simulink model "spectrum_analyser"  (R2020a)
settings: Solver=VariableStepAuto  StartTime=0.0  StopTime=100000/256e6  RelTol=1e-3
InitFcn:
  | fs = 256e6;
undefined symbols (not defined in the file): designMultirateFIR
libraries: hdlsllib x14, dspmlti4 x6, dspswit3 x4, simulink x3, dspsigops x2, dspsigattribs x2, slib_spectrum_analyser x1
(part 1 of 2)
settings Model: Creator=david  LastModifiedBy=kevin
settings OptimizationCC: BlockReduction=off  ConditionallyExecuteInputs=off  DefaultParameterBehavior=Inlined
settings DebuggingCC: AlgebraicLoopMsg=error
settings HardwareCC: ProdBitPerPointer=32  ProdBitPerSizeT=32  ProdBitPerPtrDiffT=32  ProdLargestAtomicFloat=None  ProdIntDivRoundTo=Undefined  ProdEndianess=Unspecified  ProdWordSize=32  ProdHWDeviceType=ASIC/FPGA->ASIC/FPGA  TargetBitPerPointer=64  TargetBitPerSizeT=64  TargetBitPerPtrDiffT=64  TargetLongLongMode=on  TargetIntDivRoundTo=Zero  TargetEndianess=LittleEndian  TargetWordSize=64  TargetHWDeviceType=Custom Processor->MATLAB Host Computer  ProdEqTarget=off

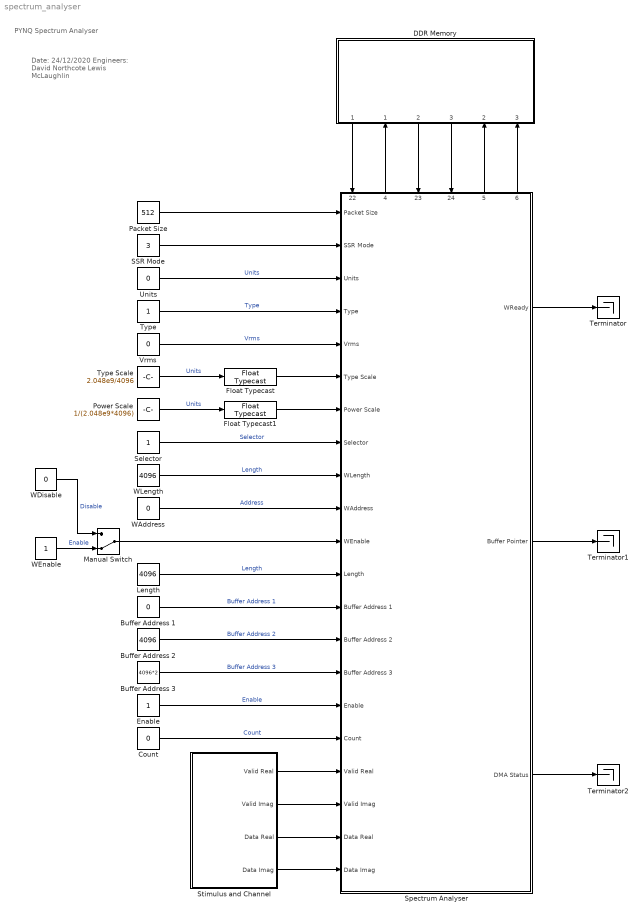
== system spectrum_analyser ==
  note: Date:		24/12/2020
      | Engineers:	David Northcote
      | 			Lewis McLaughlin
  note: PYNQ Spectrum Analyser
  Buffer Address 1 : Constant  Value=0  OutDataTypeStr=uint32  SampleTime=1/fs
  Buffer Address 2 : Constant  Value=4096  OutDataTypeStr=uint32  SampleTime=1/fs
  Buffer Address 3 : Constant  Value=4096*2  OutDataTypeStr=uint32  SampleTime=1/fs
  Count : Constant  Value=0  OutDataTypeStr=uint32  SampleTime=1/fs
  DDR Memory : Subsystem
      settings: PortSchema="{\"entries\":[{\"content\":{\"sides\":[{\"content\":{\"connectorIds\":[]},\"type\":\"ConnectorPlacement.EquallySpacedRectSide\",\"uuid\":\"d9e4a1d3-1a90-455f-8481-c9ba23695512\"},{\"content\":{\"connectorIds\":[],\"side\":\"RIGHT\"},\"type\":\"ConnectorPlacement.EquallySpacedRectSide\",\"uuid\":\"d5cbf6c4-ca28-4b6e-a385-26c8d45a1027\"},{\"content\":{\"connectorIds\":[],\"side\":\"TOP\"},\"type\":\"ConnectorPlacement.EquallySpacedRectSide\",\"uuid\":\"1f61d25a-c781-4c7b-9600-adf853a1e7e2\"},{\"content\":{\"connectorIds\":[\"Out1\",\"In1\",\"Out2\",\"Out3\",\"In2\",\"In3\"],\"side\":\"BOTTOM\"},\"type\":\"ConnectorPlacement.EquallySpacedRectSide\",\"uuid\":\"b1131089-25c6-4639-a5ae-8f8dd9cc5fb0\"}]},\"type\":\"ConnectorPlacement.EquallySpacedConnector\",\"uuid\":\"baa6cdf8-4ad4-4b76-ad8b-23012dfe0a1e\"}],\"packageUris\":[\"http://schema.mathworks.com/mf0/Connector/19700101\"],\"version\":\"1.0\"}"
  Enable : Constant  OutDataTypeStr=uint32  SampleTime=1/fs
  Float Typecast : FloatTypecast
  Float Typecast1 : FloatTypecast
  Length : Constant  Value=4096  OutDataTypeStr=uint32  SampleTime=1/fs
  Manual Switch : ManualSwitch  CurrentSetting=0
  Packet Size : Constant  Value=512  OutDataTypeStr=uint32  SampleTime=-1
  Power Scale : Constant  Value=1/(2.048e9*4096)  OutDataTypeStr=single  SampleTime=-1
  SSR Mode : Constant  Value=3  OutDataTypeStr=uint32  SampleTime=-1
  Selector : Constant  OutDataTypeStr=uint32  SampleTime=-1
  Spectrum Analyser : Subsystem  TreatAsAtomicUnit=on
      settings: PortSchema="{\"entries\":[{\"content\":{\"sides\":[{\"content\":{\"connectorIds\":[\"In1\",\"In2\",\"In3\",\"In4\",\"In5\",\"In6\",\"In7\",\"In8\",\"In9\",\"In10\",\"In11\",\"In12\",\"In13\",\"In14\",\"In15\",\"In16\",\"In17\",\"In18\",\"In19\",\"In20\",\"In21\"]},\"type\":\"ConnectorPlacement.EquallySpacedRectSide\",\"uuid\":\"cc2cc642-11de-4ac0-af05-03fa45094956\"},{\"content\":{\"connectorIds\":[\"Out1\",\"Out2\",\"Out3\"],\"side\":\"RIGHT\"},\"type\":\"ConnectorPlacement.EquallySpacedRectSide\",\"uuid\":\"6db9fe89-3396-451d-908f-f3a7c837a938\"},{\"content\":{\"connectorIds\":[\"In22\",\"Out4\",\"In23\",\"In24\",\"Out5\",\"Out6\"],\"side\":\"TOP\"},\"type\":\"ConnectorPlacement.EquallySpacedRectSide\",\"uuid\":\"bd53c193-ffde-49a5-ab31-00011bb85ae9\"}]},\"type\":\"ConnectorPlacement.EquallySpacedConnector\",\"uuid\":\"7a597bb5-a924-4306-9058-810ed9aba18e\"}],\"packageUris\":[\"http://schema.mathworks.com/mf0/Connector/19700101\"],\"version\":\"1.0\"}"
  Stimulus and Channel : Subsystem
  Terminator : Terminator
  Terminator1 : Terminator
  Terminator2 : Terminator
  Type : Constant  OutDataTypeStr=uint32  SampleTime=-1
  Type Scale : Constant  Value=2.048e9/4096  OutDataTypeStr=single  SampleTime=-1
  Units : Constant  Value=0  OutDataTypeStr=uint32  SampleTime=-1
  Vrms : Constant  Value=0  OutDataTypeStr=uint32  SampleTime=-1
  WAddress : Constant  Value=0  OutDataTypeStr=uint32  SampleTime=1/fs
  WDisable : Constant  Value=0  OutDataTypeStr=uint32  SampleTime=1/fs
  WEnable : Constant  OutDataTypeStr=uint32  SampleTime=1/fs
  WLength : Constant  Value=4096  OutDataTypeStr=uint32  SampleTime=1/fs
  wires:
  Stimulus and Channel/1(Valid Real) -> Spectrum Analyser/18(Valid Real)
  Stimulus and Channel/2(Valid Imag) -> Spectrum Analyser/19(Valid Imag)
  Stimulus and Channel/3(Data Real) -> Spectrum Analyser/20(Data Real)
  Stimulus and Channel/4(Data Imag) -> Spectrum Analyser/21(Data Imag)
  Vrms/1 -> Spectrum Analyser/5(Vrms)  "Vrms"
  Type/1 -> Spectrum Analyser/4(Type)  "Type"
  Units/1 -> Spectrum Analyser/3(Units)  "Units"
  Type Scale/1 -> Float Typecast/1  "Units"
  Float Typecast/1 -> Spectrum Analyser/6(Type Scale)
  Float Typecast1/1 -> Spectrum Analyser/7(Power Scale)
  Power Scale/1 -> Float Typecast1/1  "Units"
  Selector/1 -> Spectrum Analyser/8(Selector)  "Selector"
  SSR Mode/1 -> Spectrum Analyser/2(SSR Mode)
  Packet Size/1 -> Spectrum Analyser/1(Packet Size)
  WEnable/1 -> Manual Switch/2  "Enable"
  WDisable/1 -> Manual Switch/1  "Disable"
  Manual Switch/1 -> Spectrum Analyser/11(WEnable)
  WAddress/1 -> Spectrum Analyser/10(WAddress)  "Address"
  WLength/1 -> Spectrum Analyser/9(WLength)  "Length"
  Spectrum Analyser/4(axim_rd_m2s) -> DDR Memory/1(axim_rd_m2s)
  Spectrum Analyser/5(axim_wr_m2s) -> DDR Memory/2(axim_wr_m2s)
  Spectrum Analyser/6(axim_wr_data) -> DDR Memory/3(axim_wr_data)
  DDR Memory/1(axim_rd_s2m) -> Spectrum Analyser/22(axim_rd_s2m)
  DDR Memory/2(axim_rd_data) -> Spectrum Analyser/23(axim_rd_data)
  DDR Memory/3(axim_wr_s2m) -> Spectrum Analyser/24(axim_wr_s2m)
  Length/1 -> Spectrum Analyser/12(Length)  "Length"
  Buffer Address 1/1 -> Spectrum Analyser/13(Buffer Address 1)  "Buffer Address 1"
  Buffer Address 3/1 -> Spectrum Analyser/15(Buffer Address 3)  "Buffer Address 3"
  Buffer Address 2/1 -> Spectrum Analyser/14(Buffer Address 2)  "Buffer Address 2"
  Enable/1 -> Spectrum Analyser/16(Enable)  "Enable"
  Count/1 -> Spectrum Analyser/17(Count)  "Count"
  Spectrum Analyser/1(WReady) -> Terminator/1
  Spectrum Analyser/2(Buffer Pointer) -> Terminator1/1
  Spectrum Analyser/3(DMA Status) -> Terminator2/1

== system spectrum_analyser/DDR Memory ==
  axim_rd_m2s : Inport
  axim_wr_m2s : Inport  Port=2
  axim_wr_data : Inport  Port=3
  AXI Read Interface Response Model : Subsystem
      settings: PortSchema="{\"entries\":[{\"content\":{\"sides\":[{\"content\":{\"connectorIds\":[]},\"type\":\"ConnectorPlacement.EquallySpacedRectSide\",\"uuid\":\"2b557e1e-8026-43d3-80e6-d6d80e534d60\"},{\"content\":{\"connectorIds\":[\"Out1\",\"In1\",\"Out2\"],\"side\":\"RIGHT\"},\"type\":\"ConnectorPlacement.EquallySpacedRectSide\",\"uuid\":\"d37ff7b5-bcab-46eb-bf2f-7b890d421095\"},{\"content\":{\"connectorIds\":[],\"side\":\"TOP\"},\"type\":\"ConnectorPlacement.EquallySpacedRectSide\",\"uuid\":\"b7392330-958c-44c2-9b9d-e2e6efc00005\"}]},\"type\":\"ConnectorPlacement.EquallySpacedConnector\",\"uuid\":\"d6fedbd7-9a1a-42de-85f8-78943e8230da\"}],\"packageUris\":[\"http://schema.mathworks.com/mf0/Connector/19700101\"],\"version\":\"1.0\"}"
  AXI Write Interface Response Model : Subsystem
      settings: PortSchema="{\"entries\":[{\"content\":{\"sides\":[{\"content\":{\"connectorIds\":[]},\"type\":\"ConnectorPlacement.EquallySpacedRectSide\",\"uuid\":\"6953abbe-a6d5-4686-b276-b89fe5e6bb23\"},{\"content\":{\"connectorIds\":[],\"side\":\"RIGHT\"},\"type\":\"ConnectorPlacement.EquallySpacedRectSide\",\"uuid\":\"539ff6ac-c243-4534-87d0-888ff9534a8b\"},{\"content\":{\"connectorIds\":[],\"side\":\"TOP\"},\"type\":\"ConnectorPlacement.EquallySpacedRectSide\",\"uuid\":\"8a126ba7-8eec-4733-ae4d-1ac2504ae558\"},{\"content\":{\"connectorIds\":[\"Out1\",\"In1\",\"In2\"],\"side\":\"BOTTOM\"},\"type\":\"ConnectorPlacement.EquallySpacedRectSide\",\"uuid\":\"05254abb-7168-4864-8cc1-53a55061df5a\"}]},\"type\":\"ConnectorPlacement.EquallySpacedConnector\",\"uuid\":\"821e8dd7-bdc5-437f-b697-1dcc78127ace\"}],\"packageUris\":[\"http://schema.mathworks.com/mf0/Connector/19700101\"],\"version\":\"1.0\"}"
  axim_rd_s2m : Outport
  axim_rd_data : Outport  Port=2
  axim_wr_s2m : Outport  Port=3
  wires:
  axim_wr_m2s/1 -> AXI Write Interface Response Model/1(axim_wr_m2s)
  AXI Read Interface Response Model/1(axim_rd_data) -> axim_rd_data/1  "axim_rd_data"
  AXI Write Interface Response Model/1(axim_wr_s2m) -> axim_wr_s2m/1
  axim_rd_m2s/1 -> AXI Read Interface Response Model/1(axim_rd_m2s)
  AXI Read Interface Response Model/2(axim_rd_s2m) -> axim_rd_s2m/1  "axim_rd_s2m"
  axim_wr_data/1 -> AXI Write Interface Response Model/2(axim_wr_data)

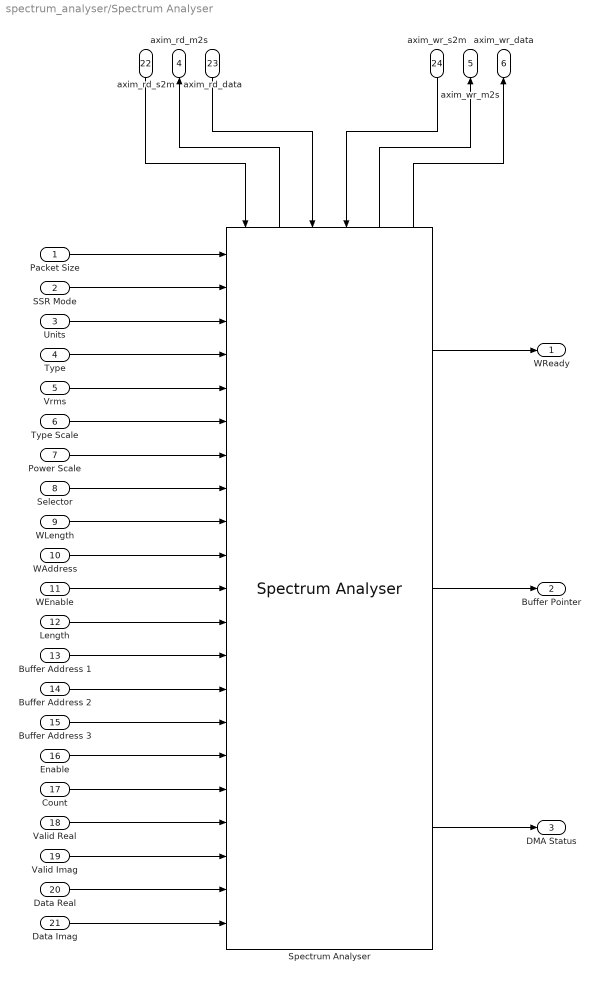
== system spectrum_analyser/Spectrum Analyser ==
  Packet Size : Inport
  SSR Mode : Inport  Port=2
  Units : Inport  Port=3
  Type : Inport  Port=4
  Vrms : Inport  Port=5
  Type Scale : Inport  Port=6
  Power Scale : Inport  Port=7
  Selector : Inport  Port=8
  WLength : Inport  Port=9
  WAddress : Inport  Port=10
  WEnable : Inport  Port=11
  Length : Inport  Port=12
  Buffer Address 1 : Inport  Port=13
  Buffer Address 2 : Inport  Port=14
  Buffer Address 3 : Inport  Port=15
  Enable : Inport  Port=16
  Count : Inport  Port=17
  Valid Real : Inport  Port=18
  Valid Imag : Inport  Port=19
  Data Real : Inport  Port=20
  Data Imag : Inport  Port=21
  axim_rd_s2m : Inport  Port=22
  axim_rd_data : Inport  Port=23
  axim_wr_s2m : Inport  Port=24
  Spectrum Analyser : slib_spectrum_analyser/Spectrum Analyser  SystemSampleTime=-1  Latency=0  AutoFrameSizeCalculation=off
      settings: PortSchema="{\"entries\":[{\"content\":{\"sides\":[{\"content\":{\"connectorIds\":[\"In1\",\"In2\",\"In3\",\"In4\",\"In5\",\"In6\",\"In7\",\"In8\",\"In9\",\"In10\",\"In11\",\"In12\",\"In13\",\"In14\",\"In15\",\"In16\",\"In17\",\"In18\",\"In19\",\"In20\",\"In21\"]},\"type\":\"ConnectorPlacement.EquallySpacedRectSide\",\"uuid\":\"d853649d-72ce-4bc9-937e-6765c6958e4b\"},{\"content\":{\"connectorIds\":[\"Out1\",\"Out2\",\"Out3\"],\"side\":\"RIGHT\"},\"type\":\"ConnectorPlacement.EquallySpacedRectSide\",\"uuid\":\"8ee09e61-17e3-46fa-8063-dedf2b48f93c\"},{\"content\":{\"connectorIds\":[\"In22\",\"Out4\",\"In23\",\"In24\",\"Out5\",\"Out6\"],\"side\":\"TOP\"},\"type\":\"ConnectorPlacement.EquallySpacedRectSide\",\"uuid\":\"c9845971-679e-4c10-9868-9337bdd39c3c\"}]},\"type\":\"ConnectorPlacement.EquallySpacedConnector\",\"uuid\":\"5955e85d-b605-4825-a1fe-b5d4f394d259\"}],\"packageUris\":[\"http://schema.mathworks.com/mf0/Connector/19700101\"],\"version\":\"1.0\"}"
  WReady : Outport
  Buffer Pointer : Outport  Port=2
  DMA Status : Outport  Port=3
  axim_rd_m2s : Outport  Port=4
  axim_wr_m2s : Outport  Port=5
  axim_wr_data : Outport  Port=6
  wires:
  Packet Size/1 -> Spectrum Analyser/1
  SSR Mode/1 -> Spectrum Analyser/2
  Units/1 -> Spectrum Analyser/3
  Type/1 -> Spectrum Analyser/4
  Vrms/1 -> Spectrum Analyser/5
  Type Scale/1 -> Spectrum Analyser/6
  Power Scale/1 -> Spectrum Analyser/7
  Selector/1 -> Spectrum Analyser/8
  WLength/1 -> Spectrum Analyser/9
  WAddress/1 -> Spectrum Analyser/10
  WEnable/1 -> Spectrum Analyser/11
  Length/1 -> Spectrum Analyser/12
  Buffer Address 1/1 -> Spectrum Analyser/13
  Buffer Address 2/1 -> Spectrum Analyser/14
  Buffer Address 3/1 -> Spectrum Analyser/15
  Enable/1 -> Spectrum Analyser/16
  Count/1 -> Spectrum Analyser/17
  Valid Real/1 -> Spectrum Analyser/18
  Valid Imag/1 -> Spectrum Analyser/19
  Data Real/1 -> Spectrum Analyser/20
  Data Imag/1 -> Spectrum Analyser/21
  axim_rd_s2m/1 -> Spectrum Analyser/22
  axim_rd_data/1 -> Spectrum Analyser/23
  axim_wr_s2m/1 -> Spectrum Analyser/24
  Spectrum Analyser/1 -> WReady/1
  Spectrum Analyser/2 -> Buffer Pointer/1
  Spectrum Analyser/3 -> DMA Status/1
  Spectrum Analyser/4 -> axim_rd_m2s/1
  Spectrum Analyser/5 -> axim_wr_m2s/1
  Spectrum Analyser/6 -> axim_wr_data/1

== system spectrum_analyser/Stimulus and Channel ==
  Channel : Subsystem
  Enable : Constant  OutDataTypeStr=boolean  SampleTime=-1
  Transmitter : Subsystem  TreatAsAtomicUnit=on
  Value : Constant  Value=hex2dec('7FFF7FFF')  OutDataTypeStr=uint32  SampleTime=-1
  Valid Real : Outport
  Valid Imag : Outport  Port=2
  Data Real : Outport  Port=3
  Data Imag : Outport  Port=4
  wires:
  Enable/1 -> Transmitter/1(Enable)  "Enable"
  Transmitter/1(Valid) -> Channel/1(Valid)
  Transmitter/2(Data) -> Channel/2(Data)
  Value/1 -> Transmitter/2(Value)  "Value"
  Channel/3(Valid Imag) -> Valid Imag/1
  Channel/4(Data Imag) -> Data Imag/1
  Channel/1(Valid Real) -> Valid Real/1
  Channel/2(Data Real) -> Data Real/1

== system spectrum_analyser/DDR Memory/AXI Read Interface Response Model ==
  axim_rd_m2s : Inport
  Bus Creator : BusCreator  Inputs=2
  Bus Selector : BusSelector  OutputSignals=rd_addr,rd_len,rd_avalid
  Constant3 : Constant  OutDataTypeStr=boolean  SampleTime=-1
  DDR : Subsystem  mask{DDR_DATA=uint16(ones(1,4096)*2^15)}
      mask init:
      | %load('ram_data');
  axim_rd_data : Outport  VectorParamsAs1DForOutWhenUnconnected=off
  axim_rd_s2m : Outport  Port=2  VectorParamsAs1DForOutWhenUnconnected=off
  wires:
  Bus Selector/2 -> DDR/2(rd_len)  "<rd_len>"
  DDR/2(rd_aready) -> Bus Creator/1  "rd_aready"
  Bus Selector/3 -> DDR/3(rd_avalid)  "<rd_avalid>"
  axim_rd_m2s/1 -> Bus Selector/1
  Bus Selector/1 -> DDR/1(rd_addr)  "<rd_addr>"
  Constant3/1 -> DDR/4(rd_ready)
  DDR/3(rd_dvalid) -> Bus Creator/2  "rd_dvalid"
  DDR/1(rd_data) -> axim_rd_data/1  "rd_data"
  Bus Creator/1 -> axim_rd_s2m/1

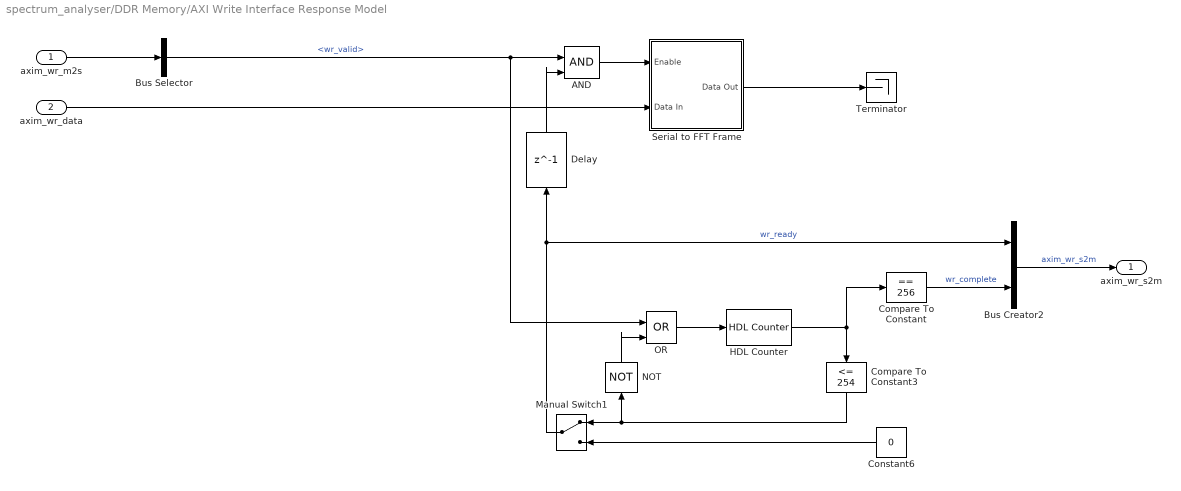
== system spectrum_analyser/DDR Memory/AXI Write Interface Response Model ==
  axim_wr_m2s : Inport
  axim_wr_data : Inport  Port=2
  AND : Logic  IconShape=distinctive  AllPortsSameDT=off  OutDataTypeStr=boolean
  Bus Creator2 : BusCreator  Inputs=2
  Bus Selector : BusSelector  OutputSignals=wr_valid
  Compare To Constant : simulink/Logic and Bit Operations/Compare To Constant  relop===  const=256  OutDataTypeStr=boolean
  Compare To Constant3 : simulink/Logic and Bit Operations/Compare To Constant  relop=<=  const=254  OutDataTypeStr=boolean
  Constant6 : Constant  Value=0  OutDataTypeStr=boolean  SampleTime=-1
  Delay : Delay  DelayLength=1  InitialCondition=0  UseCircularBuffer=on
  HDL Counter : hdlsllib/Sources/HDL Counter  CountType=Count limited  CountInit=0  CountStep=1  CountMax=256  CountFromType=Initial value  CountFrom=0  CountResetPort=off  CountLoadPort=off  CountEnbPort=on  CountDirPort=off  CountDataType=Unsigned  CountWordLen=10  CountFracLen=0  CountSampTime=1
  Manual Switch1 : ManualSwitch
  NOT : Logic  Operator=NOT  IconShape=distinctive  AllPortsSameDT=off  OutDataTypeStr=boolean
  OR : Logic  Operator=OR  IconShape=distinctive  AllPortsSameDT=off  OutDataTypeStr=boolean
  Serial to FFT Frame : Subsystem  mask{N=4096}
      mask prompts: N "FFT Size:"
      mask DialogControl DescGroupVar Prompt: Serial to FFT Frame
      mask DialogControl DescTextVar Prompt: This block converts serial FFT data to a frame of FFT data. An FFT shift is applied to correct for out of order FFT data.
      mask DialogControl ParameterGroupVar Prompt: Main
  Terminator : Terminator
  axim_wr_s2m : Outport
  wires:
  Delay/1 -> AND/2
  Compare To Constant/1 -> Bus Creator2/2  "wr_complete"
  Bus Selector/1 -> AND/1, OR/1  "<wr_valid>"
  AND/1 -> Serial to FFT Frame/1(Enable)
  Constant6/1 -> Manual Switch1/2
  HDL Counter/1 -> Compare To Constant3/1, Compare To Constant/1
  Compare To Constant3/1 -> NOT/1, Manual Switch1/1
  OR/1 -> HDL Counter/1
  NOT/1 -> OR/2
  Bus Creator2/1 -> axim_wr_s2m/1  "axim_wr_s2m"
  Manual Switch1/1 -> Bus Creator2/1, Delay/1  "wr_ready"
  axim_wr_m2s/1 -> Bus Selector/1
  Serial to FFT Frame/1(Data Out) -> Terminator/1
  axim_wr_data/1 -> Serial to FFT Frame/2(Data In)

== system spectrum_analyser/Stimulus and Channel/Channel ==
  Valid : Inport
  Data : Inport  Port=2
  RF-ADC : Subsystem  mask{fs_ghz=4.096, decim=2x, ssr=8, mode=Fine, fc=0.256, fph=0, fcoarse=fs/4}
      mask prompts: fs_ghz "Sample Rate (GHz):"; decim "Interpolation Mode:"; ssr "Samples per AXI4-Stream Cycle:"; mode "Mixer Type:"; fc "NCO Frequency (GHz):"; fph "NCO Phase (Rads):"; fcoarse "Frequency:"
      mask init:
      | % Obtain the sample rate in Hz
      | fs = str2double(get_param(gcb, 'fs_ghz'))*1e9;
      | 
      | % Set the mode of the RF-DAC interpolation filter
      | switch get_param(gcb, 'decim')
      |     case '1x'
      |         D = 1;
      |     case '2x'
      |         D = 2;
      |     case '4x'
      |         D = 4;
      |     case '8x'
      |         D = 8;
      |     otherwise
      |         D = 1;
      | end
      | 
      | % Get the AXI-Stream clock for display to user
      | axi_clk = (fs/(str2double(get_param(gcb, 'ssr'))*D))*1e-6;
      | 
      | % Get the block mask object to manipulate settings
      | mo = get_param(gcb, 'MaskObject');
      | 
      | % Update text to display the required AXI-Stream clock
      | tc = mo.getDialogControl('axi_text');
      | tc.Prompt = ['      Required AXI-Stream Clock: ', num2str(axi_clk), ' MHz'];
      | 
      | % Set the RF-DAC Mixer mode
      | switch get_param(gcb, 'mode')
      |     case 'Bypass'
      |         m = 0;
      |     case 'Coarse'
      |         m = 1;
      |     case 'Fine'
      |         m = 2;
      |     otherwise
      |         m = 0;
      | end
      | 
      | % Set the RF-DAC Coarse Mixer mode
      | switch get_param(gcb, 'fcoarse')
      |     case 'fs/2'
      |         mc = 0;
      |     case 'fs/4'
      |         mc = 1;
      |     case '-fs/4'
      |         mc = 2;
      |     otherwise
      |         mc = 0;
      | end
      | 
      | % Set other blocks
      | set_param([gcb, '/Decimation Filter'], 'decim', get_param(gcb, 'decim'));
      mask Callback fs_ghz:
      | % Obtain the sample rate in Hz
      | fs = str2double(get_param(gcb, 'fs_ghz'))*1e9;
      | 
      | % Set the mode of the RF-DAC interpolation filter
      | switch get_param(gcb, 'decim')
      |     case '1x'
      |         D = 1;
      |     case '2x'
      |         D = 2;
      |     case '4x'
      |         D = 4;
      |     case '8x'
      |         D = 8;
      |     otherwise
      |         D = 1;
      | end
      | 
      | % Get the AXI-Stream clock for display to user
      | axi_clk = (fs/(str2double(get_param(gcb, 'ssr'))*D))*1e-6;
      | 
      | % Get the block mask object to manipulate settings
      | mo = get_param(gcb, 'MaskObject');
      | 
      | % Update text to display the required AXI-Stream clock
      | tc = mo.getDialogControl('axi_text');
      | tc.Prompt = ['      Required AXI-Stream Clock: ', num2str(axi_clk), ' MHz'];
      mask TypeOptions decim: 1x | 2x | 4x | 8x
      mask Callback decim:
      | % Obtain the sample rate in Hz
      | fs = str2double(get_param(gcb, 'fs_ghz'))*1e9;
      | 
      | % Set the mode of the RF-DAC interpolation filter
      | switch get_param(gcb, 'decim')
      |     case '1x'
      |         D = 1;
      |     case '2x'
      |         D = 2;
      |     case '4x'
      |         D = 4;
      |     case '8x'
      |         D = 8;
      |     otherwise
      |         D = 1;
      | end
      | 
      | % Get the AXI-Stream clock for display to user
      | axi_clk = (fs/(str2double(get_param(gcb, 'ssr'))*D))*1e-6;
      | 
      | % Get the block mask object to manipulate settings
      | mo = get_param(gcb, 'MaskObject');
      | 
      | % Update text to display the required AXI-Stream clock
      | tc = mo.getDialogControl('axi_text');
      | tc.Prompt = ['      Required AXI-Stream Clock: ', num2str(axi_clk), ' MHz'];
      mask TypeOptions ssr: 1 | 2 | 3 | 4 | 5 | 6 | 7 | 8 | 9 | 10 | 11 | 12 | 13 | 14 | 15 | 16
      mask Callback ssr:
      | % Obtain the sample rate in Hz
      | fs = str2double(get_param(gcb, 'fs_ghz'))*1e9;
      | 
      | % Set the mode of the RF-DAC interpolation filter
      | switch get_param(gcb, 'decim')
      |     case '1x'
      |         D = 1;
      |     case '2x'
      |         D = 2;
      |     case '4x'
      |         D = 4;
      |     case '8x'
      |         D = 8;
      |     otherwise
      |         D = 1;
      | end
      | 
      | % Get the AXI-Stream clock for display to user
      | axi_clk = (fs/(str2double(get_param(gcb, 'ssr'))*D))*1e-6;
      | 
      | % Get the block mask object to manipulate settings
      | mo = get_param(gcb, 'MaskObject');
      | 
      | % Update text to display the required AXI-Stream clock
      | tc = mo.getDialogControl('axi_text');
      | tc.Prompt = ['      Required AXI-Stream Clock: ', num2str(axi_clk), ' MHz'];
      mask TypeOptions mode: Coarse | Fine
      mask Callback mode:
      | % Get the block mask object to manipulate settings
      | mo = get_param(gcb, 'MaskObject');
      | 
      | % Hide group depending on Mixer mode choice
      | switch get_param(gcb, 'mode')
      |     case 'Bypass'
      |         mo.getDialogControl('coarse_group').Visible='off';
      |         mo.getDialogControl('mixer_group').Visible='off';
      |     case 'Coarse'
      |         mo.getDialogControl('coarse_group').Visible='on';
      |         mo.getDialogControl('mixer_group').Visible='off';
      |     case 'Fine'
      |         mo.getDialogControl('coarse_group').Visible='off';
      |         mo.getDialogControl('mixer_group').Visible='on';
      |     otherwise
      |         mo.getDialogControl('coarse_group').Visible='off';
      |         mo.getDialogControl('mixer_group').Visible='off';
      | end
      mask TypeOptions fcoarse: fs/2 | fs/4 | -fs/4
      mask DialogControl DescGroupVar Prompt: RF-DAC
      mask DialogControl DescTextVar Prompt: This block simulates one RF-ADC channel.
      mask DialogControl main_group Prompt: Data Settings
      mask DialogControl axi_text Prompt: Required AXI-Stream Clock: 256 MHz
      mask DialogControl Container5 Prompt: Mixer Settings
  RF-DAC : Subsystem  mask{fs_ghz=4.096, interp=4x, ssr=4, mode=Fine, fc=0.512, fph=0, fcoarse=fs/4}
      mask prompts: fs_ghz "Sample Rate (GHz):"; interp "Interpolation Mode:"; ssr "Samples per AXI4-Stream Cycle:"; mode "Mixer Type:"; fc "NCO Frequency (GHz):"; fph "NCO Phase (Rads):"; fcoarse "Frequency:"
      mask init:
      | % Obtain the sample rate in Hz
      | fs = str2double(get_param(gcb, 'fs_ghz'))*1e9;
      | 
      | % Set the mode of the RF-DAC interpolation filter
      | switch get_param(gcb, 'interp')
      |     case '1x'
      |         L = 1;
      |     case '2x'
      |         L = 2;
      |     case '4x'
      |         L = 4;
      |     case '8x'
      |         L = 8;
      |     otherwise
      |         L = 1;
      | end
      | 
      | % Get the AXI-Stream clock for display to user
      | axi_clk = (fs/(str2double(get_param(gcb, 'ssr'))*L))*1e-6;
      | 
      | % Get the block mask object to manipulate settings
      | mo = get_param(gcb, 'MaskObject');
      | 
      | % Update text to display the required AXI-Stream clock
      | tc = mo.getDialogControl('axi_text');
      | tc.Prompt = ['      Required AXI-Stream Clock: ', num2str(axi_clk), ' MHz'];
      | 
      | % Set the RF-DAC Mixer mode
      | switch get_param(gcb, 'mode')
      |     case 'Bypass'
      |         m = 0;
      |     case 'Coarse'
      |         m = 1;
      |     case 'Fine'
      |         m = 2;
      |     otherwise
      |         m = 0;
      | end
      | 
      | % Set the RF-DAC Coarse Mixer mode
      | switch get_param(gcb, 'fcoarse')
      |     case 'fs/2'
      |         mc = 0;
      |     case 'fs/4'
      |         mc = 1;
      |     case '-fs/4'
      |         mc = 2;
      |     otherwise
      |         mc = 0;
      | end
      | 
      | % Set other blocks
      | set_param([gcb, '/Interpolation Filter'], 'interp', get_param(gcb, 'interp'));
      mask Callback fs_ghz:
      | % Obtain the sample rate in Hz
      | fs = str2double(get_param(gcb, 'fs_ghz'))*1e9;
      | 
      | % Set the mode of the RF-DAC interpolation filter
      | switch get_param(gcb, 'interp')
      |     case '1x'
      |         L = 1;
      |     case '2x'
      |         L = 2;
      |     case '4x'
      |         L = 4;
      |     case '8x'
      |         L = 8;
      |     otherwise
      |         L = 1;
      | end
      | 
      | % Get the AXI-Stream clock for display to user
      | axi_clk = (fs/(str2double(get_param(gcb, 'ssr'))*L))*1e-6;
      | 
      | % Get the block mask object to manipulate settings
      | mo = get_param(gcb, 'MaskObject');
      | 
      | % Update text to display the required AXI-Stream clock
      | tc = mo.getDialogControl('axi_text');
      | tc.Prompt = ['      Required AXI-Stream Clock: ', num2str(axi_clk), ' MHz'];
      mask TypeOptions interp: 1x | 2x | 4x | 8x
      mask Callback interp:
      | % Obtain the sample rate in Hz
      | fs = str2double(get_param(gcb, 'fs_ghz'))*1e9;
      | 
      | % Set the mode of the RF-DAC interpolation filter
      | switch get_param(gcb, 'interp')
      |     case '1x'
      |         L = 1;
      |     case '2x'
      |         L = 2;
      |     case '4x'
      |         L = 4;
      |     case '8x'
      |         L = 8;
      |     otherwise
      |         L = 1;
      | end
      | 
      | % Get the AXI-Stream clock for display to user
      | axi_clk = (fs/(str2double(get_param(gcb, 'ssr'))*L))*1e-6;
      | 
      | % Get the block mask object to manipulate settings
      | mo = get_param(gcb, 'MaskObject');
      | 
      | % Update text to display the required AXI-Stream clock
      | tc = mo.getDialogControl('axi_text');
      | tc.Prompt = ['      Required AXI-Stream Clock: ', num2str(axi_clk), ' MHz'];
      mask TypeOptions ssr: 1 | 2 | 3 | 4 | 5 | 6 | 7 | 8 | 9 | 10 | 11 | 12 | 13 | 14 | 15 | 16
      mask Callback ssr:
      | % Obtain the sample rate in Hz
      | fs = str2double(get_param(gcb, 'fs_ghz'))*1e9;
      | 
      | % Set the mode of the RF-DAC interpolation filter
      | switch get_param(gcb, 'interp')
      |     case '1x'
      |         L = 1;
      |     case '2x'
      |         L = 2;
      |     case '4x'
      |         L = 4;
      |     case '8x'
      |         L = 8;
      |     otherwise
      |         L = 1;
      | end
      | 
      | % Get the AXI-Stream clock for display to user
      | axi_clk = (fs/(str2double(get_param(gcb, 'ssr'))*L))*1e-6;
      | 
      | % Get the block mask object to manipulate settings
      | mo = get_param(gcb, 'MaskObject');
      | 
      | % Update text to display the required AXI-Stream clock
      | tc = mo.getDialogControl('axi_text');
      | tc.Prompt = ['      Required AXI-Stream Clock: ', num2str(axi_clk), ' MHz'];
      mask TypeOptions mode: Coarse | Fine
      mask Callback mode:
      | % Get the block mask object to manipulate settings
      | mo = get_param(gcb, 'MaskObject');
      | 
      | % Hide group depending on Mixer mode choice
      | switch get_param(gcb, 'mode')
      |     case 'Bypass'
      |         mo.getDialogControl('coarse_group').Visible='off';
      |         mo.getDialogControl('mixer_group').Visible='off';
      |     case 'Coarse'
      |         mo.getDialogControl('coarse_group').Visible='on';
      |         mo.getDialogControl('mixer_group').Visible='off';
      |     case 'Fine'
      |         mo.getDialogControl('coarse_group').Visible='off';
      |         mo.getDialogControl('mixer_group').Visible='on';
      |     otherwise
      |         mo.getDialogControl('coarse_group').Visible='off';
      |         mo.getDialogControl('mixer_group').Visible='off';
      | end
      mask TypeOptions fcoarse: fs/2 | fs/4 | -fs/4
      mask DialogControl DescGroupVar Prompt: RF-DAC
      mask DialogControl DescTextVar Prompt: This block simulates one RF-DAC channel.
      mask DialogControl main_group Prompt: Data Settings
      mask DialogControl axi_text Prompt: Required AXI-Stream Clock: 256 MHz
      mask DialogControl Container5 Prompt: Mixer Settings
  RX RF Balun : Gain  Gain=1/2
  TX RF Balun : Gain  Gain=1/2
  Valid Real : Outport
  Data Real : Outport  Port=2
  Valid Imag : Outport  Port=3
  Data Imag : Outport  Port=4
  wires:
  TX RF Balun/1 -> RX RF Balun/1
  Valid/1 -> RF-DAC/1(Valid)
  RF-ADC/3(Data Real) -> Data Real/1
  RX RF Balun/1 -> RF-ADC/1(Data In)
  Data/1 -> RF-DAC/2(Data)
  RF-ADC/4(Data Imag) -> Data Imag/1
  RF-ADC/1(Valid Real) -> Valid Real/1
  RF-DAC/1(Data Out) -> TX RF Balun/1
  RF-ADC/2(Valid Imag) -> Valid Imag/1

== system spectrum_analyser/Stimulus and Channel/Transmitter ==
  Enable : Inport
  Value : Inport  Port=2
  Transmitter : Subsystem  TreatAsAtomicUnit=on
  Valid : Outport
  Data : Outport  Port=2
  wires:
  Transmitter/2(Data) -> Data/1
  Transmitter/1(Valid) -> Valid/1
  Enable/1 -> Transmitter/1(Enable)
  Value/1 -> Transmitter/2(Value)

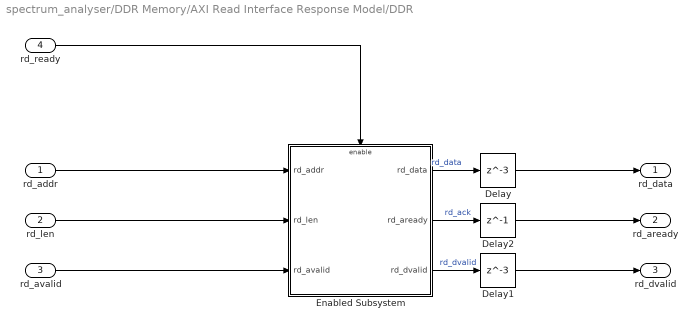
== system spectrum_analyser/DDR Memory/AXI Read Interface Response Model/DDR ==
  rd_addr : Inport
  rd_len : Inport  Port=2
  rd_avalid : Inport  Port=3
  rd_ready : Inport  Port=4
  Delay : Delay  DelayLength=3
  Delay1 : Delay  DelayLength=3
  Delay2 : Delay  DelayLength=1
  Enabled Subsystem : Subsystem  TreatAsAtomicUnit=on
  rd_data : Outport  VectorParamsAs1DForOutWhenUnconnected=off
  rd_aready : Outport  Port=2  VectorParamsAs1DForOutWhenUnconnected=off
  rd_dvalid : Outport  Port=3  VectorParamsAs1DForOutWhenUnconnected=off
  wires:
  rd_addr/1 -> Enabled Subsystem/1(rd_addr)
  rd_len/1 -> Enabled Subsystem/2(rd_len)
  Enabled Subsystem/1(rd_data) -> Delay/1  "rd_data"
  Delay/1 -> rd_data/1
  rd_avalid/1 -> Enabled Subsystem/3(rd_avalid)
  Enabled Subsystem/2(rd_aready) -> Delay2/1  "rd_ack"
  rd_ready/1 -> Enabled Subsystem/Enable
  Enabled Subsystem/3(rd_dvalid) -> Delay1/1  "rd_dvalid"
  Delay1/1 -> rd_dvalid/1
  Delay2/1 -> rd_aready/1

== system spectrum_analyser/DDR Memory/AXI Write Interface Response Model/Serial to FFT Frame ==
  Enable : Inport
  Data In : Inport  Port=2
  Enabled Subsystem2 : Subsystem  TreatAsAtomicUnit=on
  Float Typecast : FloatTypecast
  Data Out : Outport
  wires:
  Float Typecast/1 -> Data Out/1
  Data In/1 -> Enabled Subsystem2/1(Data In)
  Enable/1 -> Enabled Subsystem2/Enable
  Enabled Subsystem2/1(Data Out) -> Float Typecast/1

== system spectrum_analyser/Stimulus and Channel/Channel/RF-ADC ==
  Data In : Inport
  Complex to Real-Imag : ComplexToRealImag
  Decimation Filter : Subsystem  mask{decim=2x}
      mask prompts: decim "Decimation Factor:"
      mask init:
      | fir0 = dsp.FIRDecimator('DecimationFactor', 2,...
      |                            'CoefficientsDataType', 'Custom',...
      |                            'CustomCoefficientsDataType', numerictype([], 16, 14),...
      |                            'FullPrecisionOverride', false,...
      |                            'OutputDataType', 'Custom',...
      |                            'CustomOutputDataType', numerictype([], 16, 15),...
      |                            'Numerator', [-6, 0 54, 0, -254, 0, 1230, 2048, 1230, 0, -254, 0, 54, 0, -6]/2048);
      | fir1 = dsp.FIRDecimator('DecimationFactor', 2,...
      |                            'CoefficientsDataType', 'Custom',...
      |                            'CustomCoefficientsDataType', numerictype([], 16, 14),...
      |                            'FullPrecisionOverride', false,...
      |                            'OutputDataType', 'Custom',...
      |                            'CustomOutputDataType', numerictype([], 16, 15),...
      |                            'Numerator', [-12, 0, 84, 0, -337, 0, 1008, 0, -2693, 0, 10142, 16384, 10142, 0, -2693, 0, 1008, 0, -337, 0, 84, 0 ,-12]/16384);
      | fir2 = dsp.FIRDecimator('DecimationFactor', 2,...
      |                            'CoefficientsDataType', 'Custom',...
      |                            'CustomCoefficientsDataType', numerictype([], 16, 14),...
      |                            'FullPrecisionOverride', false,...
      |                            'OutputDataType', 'Custom',...
      |                            'CustomOutputDataType', numerictype([], 16, 15),...
      |                            'Numerator', [5, 0, -17, 0, 44, 0, -96, 0, 187, 0, -335, 0, 565, 0, -906, 0, 1401, 0, -2112, 0, 3145, 0, -4723, 0, 7415, 0, -13331, 0, 41526, 65536, 41526, 0, -13331, 0, 7415, 0, -4723, 0, 3145, 0, -2112, 0, 1401, 0, -906, 0, 565, 0, -335, 0, 187, 0, -96, 0, 44, 0, -17, 0, 5]/65536);
      | switch get_param(gcb, 'decim')
      |     case '1x'
      |         if ~strcmp(get_param([gcb, '/FIR 0'], 'Commented'), 'through')
      |             set_param([gcb, '/FIR 0'],'Commented','through');
      |         end
      |         
      |         if ~strcmp(get_param([gcb, '/FIR 1'], 'Commented'), 'through')
      |             set_param([gcb, '/FIR 1'],'Commented','through');
      |         end
      |         
      |         if ~strcmp(get_param([gcb, '/FIR 2'], 'Commented'), 'through')
      |             set_param([gcb, '/FIR 2'],'Commented','through');
      |         end
      |             
      |     case '2x'
      |         if ~strcmp(get_param([gcb, '/FIR 0'], 'Commented'), 'off')
      |             set_param([gcb, '/FIR 0'],'Commented','through');
      |         end
      |         
      |         if ~strcmp(get_param([gcb, '/FIR 1'], 'Commented'), 'through')
      |             set_param([gcb, '/FIR 1'],'Commented','through');
      |         end
      |         
      |         if ~strcmp(get_param([gcb, '/FIR 2'], 'Commented'), 'through')
      |             set_param([gcb, '/FIR 2'],'Commented','off');
      |         end
      | 
      |     case '4x'
      |         if ~strcmp(get_param([gcb, '/FIR 0'], 'Commented'), 'off')
      |             set_param([gcb, '/FIR 0'],'Commented','through');
      |         end
      |         
      |         if ~strcmp(get_param([gcb, '/FIR 1'], 'Commented'), 'off')
      |             set_param([gcb, '/FIR 1'],'Commented','off');
      |         end
      |         
      |         if ~strcmp(get_param([gcb, '/FIR 2'], 'Commented'), 'through')
      |             set_param([gcb, '/FIR 2'],'Commented','off');
      |         end
      |         
      |     case '8x'
      |         if ~strcmp(get_param([gcb, '/FIR 0'], 'Commented'), 'off')
      |             set_param([gcb, '/FIR 0'],'Commented','off');
      |         end
      |         
      |         if ~strcmp(get_param([gcb, '/FIR 1'], 'Commented'), 'off')
      |             set_param([gcb, '/FIR 1'],'Commented','off');
      |         end
      |         
      |         if ~strcmp(get_param([gcb, '/FIR 2'], 'Commented'), 'off')
      |             set_param([gcb, '/FIR 2'],'Commented','off');
      |         end
      | 
      | end
      mask TypeOptions decim: 1x | 2x | 4x | 8x
      mask DialogControl DescGroupVar Prompt: RF-DAC Interpolation Filter
      mask DialogControl DescTextVar Prompt: This block simulates the RF-DAC interpolation stage using the same coefficients stored in the interpolation filters.
      mask DialogControl ParameterGroupVar Prompt: Main
  NCO and Mixer : Subsystem
  RF-ADC : Subsystem
  SSR Converter RF-ADC : Subsystem
  Valid Real : Outport  VectorParamsAs1DForOutWhenUnconnected=off
  Valid Imag : Outport  Port=2  VectorParamsAs1DForOutWhenUnconnected=off
  Data Real : Outport  Port=3  VectorParamsAs1DForOutWhenUnconnected=off
  Data Imag : Outport  Port=4  VectorParamsAs1DForOutWhenUnconnected=off
  wires:
  SSR Converter RF-ADC/2(Valid Imag) -> Valid Imag/1
  SSR Converter RF-ADC/1(Valid Real) -> Valid Real/1
  SSR Converter RF-ADC/3(Real Out) -> Data Real/1
  SSR Converter RF-ADC/4(Imag Out) -> Data Imag/1
  Complex to Real-Imag/2 -> SSR Converter RF-ADC/2(Imag In)
  Complex to Real-Imag/1 -> SSR Converter RF-ADC/1(Real In)
  Decimation Filter/1(Data Out) -> Complex to Real-Imag/1
  Data In/1 -> RF-ADC/1(Data In)
  RF-ADC/1(Data Out) -> NCO and Mixer/1(Data In)
  NCO and Mixer/1(Data Out) -> Decimation Filter/1(Data In)

== system spectrum_analyser/Stimulus and Channel/Channel/RF-DAC ==
  Valid : Inport
  Data : Inport  Port=2
  Interpolation Filter : Subsystem  mask{interp=4x}
      mask prompts: interp "Interpolation Factor:"
      mask init:
      | fir0 = dsp.FIRInterpolator('InterpolationFactor', 2,...
      |                            'CoefficientsDataType', 'Custom',...
      |                            'CustomCoefficientsDataType', numerictype([], 16, 14),...
      |                            'FullPrecisionOverride', false,...
      |                            'OutputDataType', 'Custom',...
      |                            'CustomOutputDataType', numerictype([], 16, 15),...
      |                            'Numerator', [-6, 0 54, 0, -254, 0, 1230, 2048, 1230, 0, -254, 0, 54, 0, -6]/(2048));
      | fir1 = dsp.FIRInterpolator('InterpolationFactor', 2,...
      |                            'CoefficientsDataType', 'Custom',...
      |                            'CustomCoefficientsDataType', numerictype([], 16, 14),...
      |                            'FullPrecisionOverride', false,...
      |                            'OutputDataType', 'Custom',...
      |                            'CustomOutputDataType', numerictype([], 16, 15),...
      |                            'Numerator', [-12, 0, 84, 0, -337, 0, 1008, 0, -2693, 0, 10142, 16384, 10142, 0, -2693, 0, 1008, 0, -337, 0, 84, 0 ,-12]/(16384));
      | fir2 = dsp.FIRInterpolator('InterpolationFactor', 2,...
      |                            'CoefficientsDataType', 'Custom',...
      |                            'CustomCoefficientsDataType', numerictype([], 16, 14),...
      |                            'FullPrecisionOverride', false,...
      |                            'OutputDataType', 'Custom',...
      |                            'CustomOutputDataType', numerictype([], 16, 15),...
      |                            'Numerator', [5, 0, -17, 0, 44, 0, -96, 0, 187, 0, -335, 0, 565, 0, -906, 0, 1401, 0, -2112, 0, 3145, 0, -4723, 0, 7415, 0, -13331, 0, 41526, 65536, 41526, 0, -13331, 0, 7415, 0, -4723, 0, 3145, 0, -2112, 0, 1401, 0, -906, 0, 565, 0, -335, 0, 187, 0, -96, 0, 44, 0, -17, 0, 5]/(65536));
      | switch get_param(gcb, 'interp')
      |     case '1x'
      |         if ~strcmp(get_param([gcb, '/FIR 0'], 'Commented'), 'through')
      |             set_param([gcb, '/FIR 0'],'Commented','through');
      |         end
      |         
      |         if ~strcmp(get_param([gcb, '/FIR 1'], 'Commented'), 'through')
      |             set_param([gcb, '/FIR 1'],'Commented','through');
      |         end
      |         
      |         if ~strcmp(get_param([gcb, '/FIR 2'], 'Commented'), 'through')
      |             set_param([gcb, '/FIR 2'],'Commented','through');
      |         end
      |             
      |     case '2x'
      |         if ~strcmp(get_param([gcb, '/FIR 0'], 'Commented'), 'through')
      |             set_param([gcb, '/FIR 0'],'Commented','through');
      |         end
      |         
      |         if ~strcmp(get_param([gcb, '/FIR 1'], 'Commented'), 'through')
      |             set_param([gcb, '/FIR 1'],'Commented','through');
      |         end
      |         
      |         if ~strcmp(get_param([gcb, '/FIR 2'], 'Commented'), 'off')
      |             set_param([gcb, '/FIR 2'],'Commented','off');
      |         end
      | 
      |     case '4x'
      |         if ~strcmp(get_param([gcb, '/FIR 0'], 'Commented'), 'through')
      |             set_param([gcb, '/FIR 0'],'Commented','through');
      |         end
      |         
      |         if ~strcmp(get_param([gcb, '/FIR 1'], 'Commented'), 'off')
      |             set_param([gcb, '/FIR 1'],'Commented','off');
      |         end
      |         
      |         if ~strcmp(get_param([gcb, '/FIR 2'], 'Commented'), 'off')
      |             set_param([gcb, '/FIR 2'],'Commented','off');
      |         end
      |         
      |     case '8x'
      |         if ~strcmp(get_param([gcb, '/FIR 0'], 'Commented'), 'off')
      |             set_param([gcb, '/FIR 0'],'Commented','off');
      |         end
      |         
      |         if ~strcmp(get_param([gcb, '/FIR 1'], 'Commented'), 'off')
      |             set_param([gcb, '/FIR 1'],'Commented','off');
      |         end
      |         
      |         if ~strcmp(get_param([gcb, '/FIR 2'], 'Commented'), 'off')
      |             set_param([gcb, '/FIR 2'],'Commented','off');
      |         end
      | 
      | end
      mask TypeOptions interp: 1x | 2x | 4x | 8x
      mask DialogControl DescGroupVar Prompt: RF-DAC Interpolation Filter
      mask DialogControl DescTextVar Prompt: This block simulates the RF-DAC interpolation stage using the same coefficients stored in the interpolation filters.
      mask DialogControl ParameterGroupVar Prompt: Main
  NCO and Mixer : Subsystem
  RF-DAC : Subsystem
  SSR Converter RF-DAC : Subsystem
  Data Out : Outport  VectorParamsAs1DForOutWhenUnconnected=off
  wires:
  SSR Converter RF-DAC/1(Data Out) -> Interpolation Filter/1(Data In)
  Valid/1 -> SSR Converter RF-DAC/1(Valid)
  Data/1 -> SSR Converter RF-DAC/2(Data)
  Interpolation Filter/1(Data Out) -> NCO and Mixer/1(Data In)
  NCO and Mixer/1(Data Out) -> RF-DAC/1(Data In)
  RF-DAC/1(Data Out) -> Data Out/1

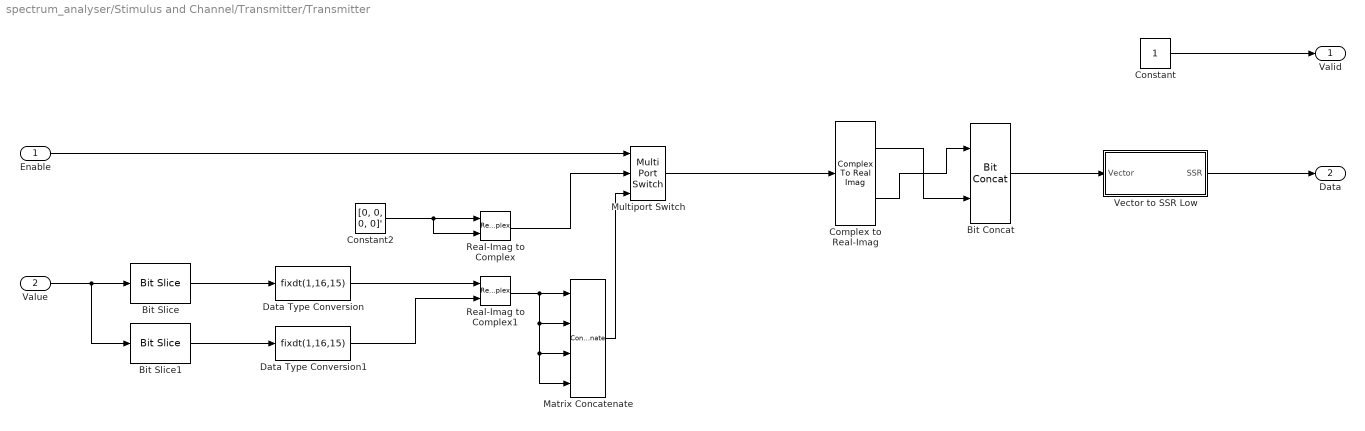
== system spectrum_analyser/Stimulus and Channel/Transmitter/Transmitter ==
  Enable : Inport
  Value : Inport  Port=2
  Bit Concat : hdlsllib/Logic and Bit Operations/Bit Concat  numInputs=2
  Bit Slice : hdlsllib/Logic and Bit Operations/Bit Slice  lidx=15  ridx=0
      settings: SourceProductBaseCode=SL
  Bit Slice1 : hdlsllib/Logic and Bit Operations/Bit Slice  lidx=31  ridx=16
      settings: SourceProductBaseCode=SL
  Complex to Real-Imag : ComplexToRealImag
  Constant : Constant  OutDataTypeStr=boolean  SampleTime=-1
  Constant2 : Constant  Value=[0, 0, 0, 0]'  VectorParams1D=off  OutDataTypeStr=fixdt(1,16,15)  SampleTime=-1
  Data Type Conversion : DataTypeConversion  OutDataTypeStr=fixdt(1,16,15)  ConvertRealWorld=Stored Integer (SI)
  Data Type Conversion1 : DataTypeConversion  OutDataTypeStr=fixdt(1,16,15)  ConvertRealWorld=Stored Integer (SI)
  Matrix Concatenate : Concatenate  NumInputs=4  Mode=Multidimensional array
  Multiport Switch : MultiPortSwitch  DataPortOrder=Zero-based contiguous  Inputs=2  zeroidx=on
  Real-Imag to Complex : RealImagToComplex
  Real-Imag to Complex1 : RealImagToComplex
  Vector to SSR Low : Subsystem  mask{N=4, hN=4}
      mask prompts: N "Samples per clock cycle:"
      mask init:
      | if ~isequal(get_param(gcb, 'N'), get_param(gcb, 'hN'))
      |     % Delete all blocks except input and output ports
      |     delete_block(setxor(setdiff(...
      |         find_system(gcb,'LookUnderMasks','on'),...
      |         {[gcb, '/Vector'], [gcb, '/SSR']}), gcb));
      | 
      |     % Delete all wires
      |     delete_line(find_system(gcb, 'FindAll', 'on', 'LookUnderMasks',...
      |         'on', 'SearchDepth', 3, 'Type', 'line', 'Connected', 'off'));
      | 
      |     % Add the bit concatenation block
      |     add_block('hdlsllib/Logic and Bit Operations/Bit Concat',...
      |         [gcb, '/Bit Concat'],...
      |         'Position', [155 55 205 330]);
      |     set_param([gcb, '/Bit Concat'], 'numInputs', num2str(N));
      | 
      |     % Add wire to output
      |     add_line(gcb, 'Bit Concat/1', 'SSR/1');
      | 
      |     % Add selector blocks and connect wires
      |     for i = 0:N-1
      |         add_block('simulink/Signal Routing/Selector',...
      |             [gcb, '/Selector', num2str(i)],...
      |             'Position', [0 82+i*90 45 128+i*90]);
      |         set_param([gcb, '/Selector', num2str(i)], 'InputPortWidth', num2str(N));
      |         set_param([gcb, '/Selector', num2str(i)], 'IndexParamArray', {num2str(N-i)});
      |         add_line(gcb, 'Vector/1', ['Selector', num2str(i), '/1'],...
      |             'autorouting', 'on');
      |         add_line(gcb, ['Selector', num2str(i), '/1'],...
      |             ['Bit Concat/', num2str(i+1)],...
      |             'autorouting', 'on');
      |     end
      |     
      |     % Set the hidden attribute to prevent unnecessary changes in
      |     % architecture while generating HDL Code.
      |     set_param(gcb, 'hN', get_param(gcb, 'N'));
      | end
      mask DialogControl DescGroupVar Prompt: Vector to SSR
      mask DialogControl DescTextVar Prompt: Convert a vector of inputs into SSR format.
  Valid : Outport
  Data : Outport  Port=2
  wires:
  Matrix Concatenate/1 -> Multiport Switch/3
  Real-Imag to Complex1/1 -> Matrix Concatenate/1, Matrix Concatenate/2, Matrix Concatenate/3, Matrix Concatenate/4
  Constant/1 -> Valid/1
  Data Type Conversion1/1 -> Real-Imag to Complex1/2
  Bit Slice1/1 -> Data Type Conversion1/1
  Bit Slice/1 -> Data Type Conversion/1
  Data Type Conversion/1 -> Real-Imag to Complex1/1
  Value/1 -> Bit Slice/1, Bit Slice1/1
  Enable/1 -> Multiport Switch/1
  Real-Imag to Complex/1 -> Multiport Switch/2
  Constant2/1 -> Real-Imag to Complex/1, Real-Imag to Complex/2
  Multiport Switch/1 -> Complex to Real-Imag/1
  Bit Concat/1 -> Vector to SSR Low/1(Vector)
  Complex to Real-Imag/1 -> Bit Concat/2
  Vector to SSR Low/1(SSR) -> Data/1
  Complex to Real-Imag/2 -> Bit Concat/1

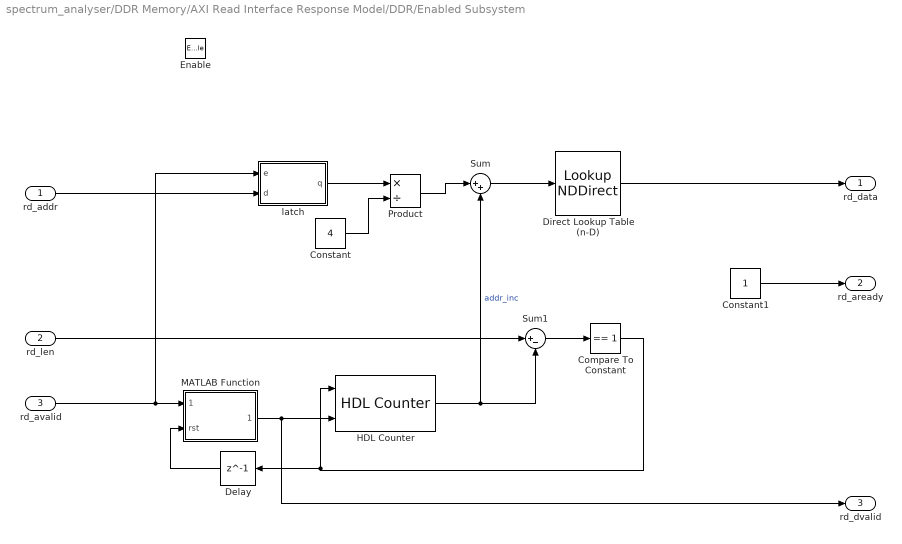
== system spectrum_analyser/DDR Memory/AXI Read Interface Response Model/DDR/Enabled Subsystem ==
  rd_addr : Inport
  rd_len : Inport  Port=2
  rd_avalid : Inport  Port=3
  Enable : EnablePort
  Compare To Constant : simulink/Logic and Bit Operations/Compare To Constant  relop===  const=1  OutDataTypeStr=boolean
  Constant : Constant  Value=4  SampleTime=-1
  Constant1 : Constant  OutDataTypeStr=boolean  SampleTime=-1
  Delay : Delay  DelayLength=1
  Direct Lookup Table (n-D) : LookupNDDirect  NumberOfTableDimensions=1  Table=DDR_DATA  DiagnosticForOutOfRangeInput=Error
  HDL Counter : hdlsllib/Sources/HDL Counter  CountType=Count limited  CountInit=0  CountStep=1  CountMax=2^16-1  CountFromType=Specify  CountFrom=0  CountResetPort=on  CountLoadPort=off  CountEnbPort=on  CountDirPort=off  CountDataType=Unsigned  CountWordLen=16  CountFracLen=0  CountSampTime=1
  MATLAB Function : MATLAB Function  TreatAsAtomicUnit=on
  Product : Product  Inputs=*/
  Sum : Sum  Inputs=|++  OutDataTypeStr=uint32
  Sum1 : Sum  Inputs=|+-
  latch : Subsystem
  rd_data : Outport  VectorParamsAs1DForOutWhenUnconnected=off
  rd_aready : Outport  Port=2  VectorParamsAs1DForOutWhenUnconnected=off
  rd_dvalid : Outport  Port=3  VectorParamsAs1DForOutWhenUnconnected=off
  wires:
  Direct Lookup Table (n-D)/1 -> rd_data/1
  HDL Counter/1 -> Sum1/2, Sum/2  "addr_inc"
  Sum1/1 -> Compare To Constant/1
  Sum/1 -> Direct Lookup Table (n-D)/1
  Compare To Constant/1 -> Delay/1, HDL Counter/1
  rd_addr/1 -> latch/2(d)
  rd_len/1 -> Sum1/1
  rd_avalid/1 -> latch/1(e), MATLAB Function/1(rd_avalid)
  MATLAB Function/1(start_counter) -> rd_dvalid/1, HDL Counter/2
  latch/1(q) -> Product/1
  Product/1 -> Sum/1
  Constant/1 -> Product/2
  Delay/1 -> MATLAB Function/2(rst)
  Constant1/1 -> rd_aready/1

== system spectrum_analyser/DDR Memory/AXI Write Interface Response Model/Serial to FFT Frame/Enabled Subsystem2 ==
  Data In : Inport
  Enable : EnablePort
  Buffer : Buffer  N=N  OutputFrames=off
  Data Out : Outport
  wires:
  Buffer/1 -> Data Out/1
  Data In/1 -> Buffer/1

== system spectrum_analyser/Stimulus and Channel/Channel/RF-ADC/Decimation Filter ==
  Data In : Inport
  FIR 0 : dspmlti4/FIR Decimation  FilterSource=Filter object  h=designMultirateFIR(1,2)  D=2  filtStruct=Direct form  FilterObject=fir0  InputProcessing=Columns as channels (frame based)  framing=Allow multirate processing  inputOffset=0  outputBufInitCond=0  roundingMode=Floor  overflowMode=off  firstCoeffDataTypeStr=Inherit: Same word length as input  firstCoeffMin=[]  firstCoeffMax=[]  firstCoeffLastDataTypeStr=Inherit: Same word length as input  outputDataTypeStr=Inherit: Same as accumulator  outputMin=[]  outputMax=[]  outputLastDataTypeStr=Inherit: Same as accumulator
  FIR 1 : dspmlti4/FIR Decimation  Commented=through  FilterSource=Filter object  h=designMultirateFIR(1,2)  D=2  filtStruct=Direct form  FilterObject=fir1  InputProcessing=Columns as channels (frame based)  framing=Allow multirate processing  inputOffset=0  outputBufInitCond=0  roundingMode=Floor  overflowMode=off  firstCoeffDataTypeStr=Inherit: Same word length as input  firstCoeffMin=[]  firstCoeffMax=[]  firstCoeffLastDataTypeStr=Inherit: Same word length as input  outputDataTypeStr=Inherit: Same as accumulator  outputMin=[]  outputMax=[]  outputLastDataTypeStr=Inherit: Same as accumulator
  FIR 2 : dspmlti4/FIR Decimation  Commented=through  FilterSource=Filter object  h=designMultirateFIR(1,2)  D=2  filtStruct=Direct form  FilterObject=fir2  InputProcessing=Columns as channels (frame based)  framing=Allow multirate processing  inputOffset=0  outputBufInitCond=0  roundingMode=Floor  overflowMode=off  firstCoeffDataTypeStr=Inherit: Same word length as input  firstCoeffMin=[]  firstCoeffMax=[]  firstCoeffLastDataTypeStr=Inherit: Same word length as input  outputDataTypeStr=Inherit: Same as accumulator  outputMin=[]  outputMax=[]  outputLastDataTypeStr=Inherit: Same as accumulator
  Data Out : Outport  VectorParamsAs1DForOutWhenUnconnected=off
  wires:
  FIR 1/1 -> FIR 2/1
  FIR 0/1 -> FIR 1/1
  Data In/1 -> FIR 0/1
  FIR 2/1 -> Data Out/1
